simulink model "Q3"  (R2019b)
settings: Solver=VariableStepAuto  StartTime=0.0  StopTime=tSim  RelTol=1e-3
values from neighbouring files (symbols this model uses):
  a0 = 0.01    [Q5.m]    (also in main3.m = 1; param3.m = -1)
  a1 = 0.2    [Q5.m]    (also in main3.m = 0; param3.m = 0)
  alpha3 = 4    [main3.m]    (also in param3.m)
  dAmp = 20    [Sol_Q1.m]    (also in main3.m = -3; param3.m = -2)
  delay = 0.5    [Sol_Q1.m]    (also in main3.m = 0; param3.m = 0.01; params2.m = 5)
  deltat = 0.01    [Q4.m]    (also in Sol_Q1.m = 0.001; main3.m; param3.m = 0.001; params2.m = 0.1)
  Gs = tf(b, [1 a])    [Q4.m]    (also in Q5.m = tf([b1 b0], [1 a1 a0]); Sol_Q1.m = tf(num, den); main3.m = tf(num, den); param3.m = tf(b, [1 a1 a0]))
  K1 = (alpha1 - a)/b    (= 1.5)    [Q4.m]    (also in Sol_Q1.m = 5; main3.m = 4; param3.m = 5)
  K2 = alpha2/b    (= 15)    [Sol_Q1.m]    (also in main3.m = 2.121; param3.m = 2.121)
  K3 = alpha3/b    (= 2)    [main3.m]    (also in param3.m)
  tauf = 0.1*tauD    (= 0.053025)    [main3.m]    (also in param3.m = 0.04242)
  tSim = 20    [Q4.m]    (also in param3.m = 10; params2.m = 400)
  umax = 8.8    [Q4.m]    (also in Sol_Q1.m = 10000; main3.m = 4.5; param3.m = 999)
  umin = -100    [Q4.m]    (also in Sol_Q1.m = -10000; main3.m = -0.9; param3.m = -999)
settings Model: Creator=adityaaaap  LastModifiedBy=adityaaaap

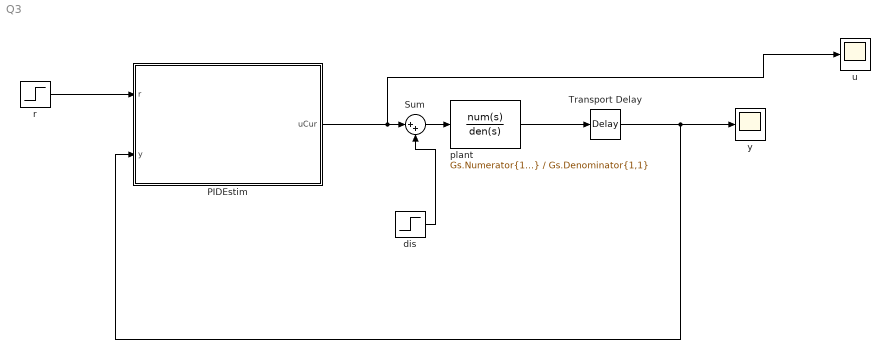
== system Q3 ==
  PIDEstim : MATLAB Function  TreatAsAtomicUnit=on
  Sum : Sum  Inputs=|++
  Transport Delay : TransportDelay  DelayTime=delay
  dis : Step  Time=tSim/2  After=dAmp  SampleTime=0
  plant : TransferFcn  Numerator=Gs.Numerator{1,1}  Denominator=Gs.Denominator{1,1}
  r : Step  Time=0  SampleTime=0
  u : Scope
  "y " : Scope
  wires:
  Sum/1 -> plant/1
  dis/1 -> Sum/2
  plant/1 -> Transport Delay/1
  PIDEstim/1(uCur) -> u/1, Sum/1
  Transport Delay/1 -> "y "/1, PIDEstim/2(y)
  r/1 -> PIDEstim/1(r)

== matlab function Q3/PIDEstim ==
  settings: updateMethod=DISCRETE  sampleTime=deltat
  data: uCur output; r input; y input; K1 parameter; K2 parameter; K3 parameter; tauf parameter; alpha3 parameter; a1 parameter; a0 parameter; deltat parameter; umin parameter; umax parameter
function uCur = PIDEstFD(r,y,K1,K2,K3,tauf,alpha3,a1,a0,deltat,umin,umax)
persistent zhat
if isempty(zhat)
    zhat=0;
end
persistent ydfpast
if isempty(ydfpast)
    ydfpast=0;
end
persistent ypast
if isempty(ypast)
    ypast=0;
end


% ndmax=100; 
% persistent(udelay)
% if isempty(udelay)
%     udelay=zeros(1,ndmax);
% end   
%estimator based MATLAB function with anti-windup
ydf=tauf/(tauf+deltat)*ydfpast+1/(tauf+deltat)*(y-ypast); 
dhat=zhat+K3*ydf;   
uCur= -K1*(y-r)-K2*ydf-dhat;
if (uCur>umax) uCur=umax;end
if (uCur<umin) uCur=umin;end
zhat=zhat-deltat*alpha3*zhat+deltat*(K3*(a1-alpha3)*ydf+K3*a0*(y-r)-alpha3*uCur);
ypast=y;
ydfpast=ydf;
%udelay=[uCur udelay(1,1:ndmax-1)];
